simulink model "carry_skip_adder"  (R2022b)
settings: Solver=FixedStepDiscrete  StartTime=0.0  StopTime=10.0  RelTol=1e-3
PreLoadFcn:
  | addpath('C:\Course_Material\UofT\ECE1718\assignment2\matlab_tests\hdlimport\carry_skip_adder');
libraries: simulink x240, hdlsllib x97
(part 1 of 2)
CloseFcn:
  | addpath('C:\Course_Material\UofT\ECE1718\assignment2\matlab_tests\hdlimport\carry_skip_adder');
  | rmpath('C:\Course_Material\UofT\ECE1718\assignment2\matlab_tests\hdlimport\carry_skip_adder');
settings Model: DataTypeOverride=Off  Creator=13698  LastModifiedBy=13698
settings OptimizationCC: BlockReduction=off  ConditionallyExecuteInputs=off  DefaultParameterBehavior=Inlined  InheritOutputTypeSmallerThanSingle=on
settings DebuggingCC: AlgebraicLoopMsg=error  InheritedTsInSrcMsg=none  SingleTaskRateTransMsg=error  IntegerOverflowMsg=none  IntegerSaturationMsg=none
settings HardwareCC: ProdBitPerPointer=32  ProdBitPerSizeT=32  ProdBitPerPtrDiffT=32  ProdLargestAtomicFloat=None  ProdIntDivRoundTo=Undefined  ProdEndianess=Unspecified  ProdWordSize=32  ProdHWDeviceType=ASIC/FPGA->ASIC/FPGA  TargetBitPerPointer=64  TargetBitPerSizeT=64  TargetBitPerPtrDiffT=64  TargetLongLongMode=on  TargetIntDivRoundTo=Zero  TargetEndianess=LittleEndian  TargetWordSize=64  TargetHWDeviceType=Custom Processor->MATLAB Host Computer  ProdEqTarget=off

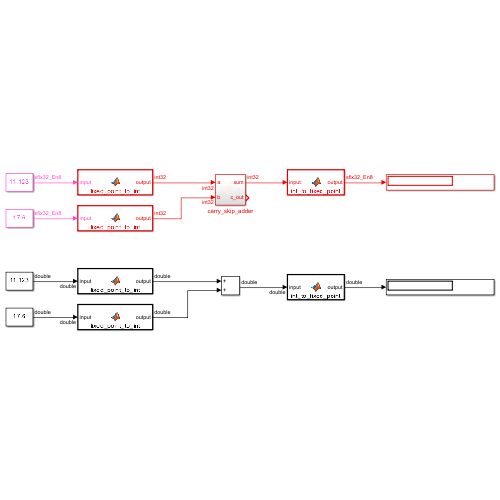
[thumbnail: Simulink's stored preview of the top-level diagram]
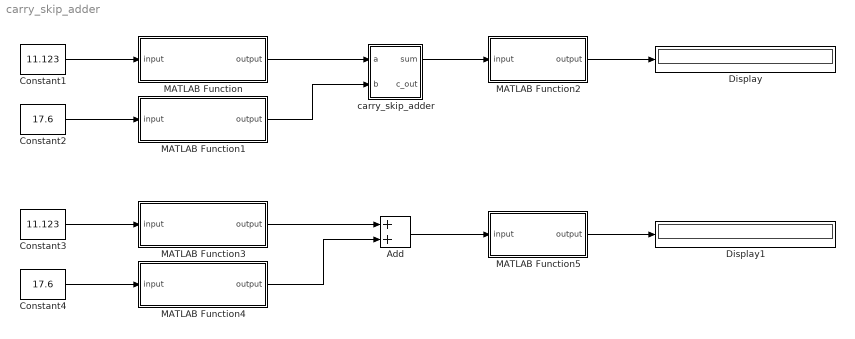
== system carry_skip_adder ==
  Add : Sum
  Constant1 : Constant  Value=11.123  OutDataTypeStr=fixdt(1,32,8)
  Constant2 : Constant  Value=17.6  OutDataTypeStr=fixdt(1,32,8)
  Constant3 : Constant  Value=11.123  OutDataTypeStr=fixdt(1,32,8)
  Constant4 : Constant  Value=17.6  OutDataTypeStr=fixdt(1,32,8)
  Display : Display
  Display1 : Display
  MATLAB Function : MATLAB Function  TreatAsAtomicUnit=on
  MATLAB Function1 : MATLAB Function  TreatAsAtomicUnit=on
  MATLAB Function2 : MATLAB Function  TreatAsAtomicUnit=on
  MATLAB Function3 : MATLAB Function  TreatAsAtomicUnit=on
  MATLAB Function4 : MATLAB Function  TreatAsAtomicUnit=on
  MATLAB Function5 : MATLAB Function  TreatAsAtomicUnit=on
  carry_skip_adder : Subsystem
  wires:
  Constant1/1 -> MATLAB Function/1(input)
  MATLAB Function/1(output) -> carry_skip_adder/1(a)
  Constant2/1 -> MATLAB Function1/1(input)
  MATLAB Function1/1(output) -> carry_skip_adder/2(b)
  carry_skip_adder/1(sum) -> MATLAB Function2/1(input)
  MATLAB Function2/1(output) -> Display/1
  MATLAB Function3/1(output) -> Add/1
  MATLAB Function4/1(output) -> Add/2
  Constant4/1 -> MATLAB Function4/1(input)
  Add/1 -> MATLAB Function5/1(input)
  Constant3/1 -> MATLAB Function3/1(input)
  MATLAB Function5/1(output) -> Display1/1

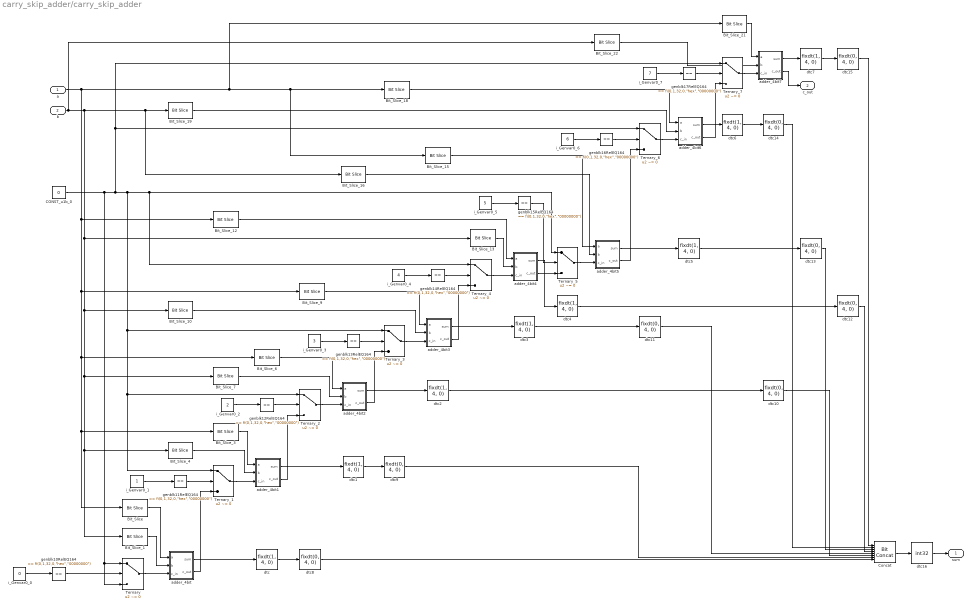
== system carry_skip_adder/carry_skip_adder ==
  a : Inport  OutDataTypeStr=int32  SampleTime=-1
  b : Inport  Port=2  OutDataTypeStr=int32  SampleTime=-1
  Bit_Slice : hdlsllib/Logic and Bit Operations/Bit Slice  lidx=double(3)  ridx=double(0)
  Bit_Slice_1 : hdlsllib/Logic and Bit Operations/Bit Slice  lidx=double(3)  ridx=double(0)
  Bit_Slice_10 : hdlsllib/Logic and Bit Operations/Bit Slice  lidx=double(15)  ridx=double(12)
  Bit_Slice_12 : hdlsllib/Logic and Bit Operations/Bit Slice  lidx=double(19)  ridx=double(16)
  Bit_Slice_13 : hdlsllib/Logic and Bit Operations/Bit Slice  lidx=double(19)  ridx=double(16)
  Bit_Slice_15 : hdlsllib/Logic and Bit Operations/Bit Slice  lidx=double(23)  ridx=double(20)
  Bit_Slice_16 : hdlsllib/Logic and Bit Operations/Bit Slice  lidx=double(23)  ridx=double(20)
  Bit_Slice_18 : hdlsllib/Logic and Bit Operations/Bit Slice  lidx=double(27)  ridx=double(24)
  Bit_Slice_19 : hdlsllib/Logic and Bit Operations/Bit Slice  lidx=double(27)  ridx=double(24)
  Bit_Slice_21 : hdlsllib/Logic and Bit Operations/Bit Slice  lidx=double(31)  ridx=double(28)
  Bit_Slice_22 : hdlsllib/Logic and Bit Operations/Bit Slice  lidx=double(31)  ridx=double(28)
  Bit_Slice_3 : hdlsllib/Logic and Bit Operations/Bit Slice  lidx=double(7)  ridx=double(4)
  Bit_Slice_4 : hdlsllib/Logic and Bit Operations/Bit Slice  lidx=double(7)  ridx=double(4)
  Bit_Slice_6 : hdlsllib/Logic and Bit Operations/Bit Slice  lidx=double(11)  ridx=double(8)
  Bit_Slice_7 : hdlsllib/Logic and Bit Operations/Bit Slice  lidx=double(11)  ridx=double(8)
  Bit_Slice_9 : hdlsllib/Logic and Bit Operations/Bit Slice  lidx=double(15)  ridx=double(12)
  CONST_u1b_0 : Constant  Value=0  OutDataTypeStr=fixdt(0, 1, 0)  SampleTime=-1
  Concat : hdlsllib/Logic and Bit Operations/Bit Concat  numInputs=8
  Ternary : Switch  Criteria=u2 ~= 0  Threshold=double(0)  OutDataTypeStr=fixdt(0, 1, 0)  SampleTime=-1  SaturateOnIntegerOverflow=off  InputSameDT=off
  Ternary_{1..7} (7 alike) : Switch  Criteria=u2 ~= 0  Threshold=double(0)  OutDataTypeStr=fixdt(0, 1, 0)  SampleTime=-1  SaturateOnIntegerOverflow=off  InputSameDT=off
  adder_4bit : Subsystem
  adder_4bit1 : Subsystem
  adder_4bit2 : Subsystem
  adder_4bit3 : Subsystem
  adder_4bit4 : Subsystem
  adder_4bit5 : Subsystem
  adder_4bit6 : Subsystem
  adder_4bit7 : Subsystem
  dtc{,1..7} (8 alike) : DataTypeConversion  OutDataTypeStr=fixdt(1, 4, 0)  SampleTime=-1  SaturateOnIntegerOverflow=off  RndMeth=Floor
  dtc{8..15} (8 alike) : DataTypeConversion  OutDataTypeStr=fixdt(0, 4, 0)  ConvertRealWorld=Stored Integer (SI)  SampleTime=-1  SaturateOnIntegerOverflow=off  RndMeth=Floor
  dtc16 : DataTypeConversion  OutDataTypeStr=int32  ConvertRealWorld=Stored Integer (SI)  SampleTime=-1  SaturateOnIntegerOverflow=off  RndMeth=Floor
  genblk10RelEQ164 : simulink/Logic and Bit Operations/Compare To Constant  relop===  const="fi(0,1,32,0,\"hex\",\"00000000\")"  OutDataTypeStr=boolean
  genblk11RelEQ164 : simulink/Logic and Bit Operations/Compare To Constant  relop===  const="fi(0,1,32,0,\"hex\",\"00000000\")"  OutDataTypeStr=boolean
  genblk12RelEQ164 : simulink/Logic and Bit Operations/Compare To Constant  relop===  const="fi(0,1,32,0,\"hex\",\"00000000\")"  OutDataTypeStr=boolean
  genblk13RelEQ164 : simulink/Logic and Bit Operations/Compare To Constant  relop===  const="fi(0,1,32,0,\"hex\",\"00000000\")"  OutDataTypeStr=boolean
  genblk14RelEQ164 : simulink/Logic and Bit Operations/Compare To Constant  relop===  const="fi(0,1,32,0,\"hex\",\"00000000\")"  OutDataTypeStr=boolean
  genblk15RelEQ164 : simulink/Logic and Bit Operations/Compare To Constant  relop===  const="fi(0,1,32,0,\"hex\",\"00000000\")"  OutDataTypeStr=boolean
  genblk16RelEQ164 : simulink/Logic and Bit Operations/Compare To Constant  relop===  const="fi(0,1,32,0,\"hex\",\"00000000\")"  OutDataTypeStr=boolean
  genblk17RelEQ164 : simulink/Logic and Bit Operations/Compare To Constant  relop===  const="fi(0,1,32,0,\"hex\",\"00000000\")"  OutDataTypeStr=boolean
  i_Genvar0_0 : Constant  Value=0  OutDataTypeStr=int32  SampleTime=-1
  i_Genvar0_1 : Constant  OutDataTypeStr=int32  SampleTime=-1
  i_Genvar0_2 : Constant  Value=2  OutDataTypeStr=int32  SampleTime=-1
  i_Genvar0_3 : Constant  Value=3  OutDataTypeStr=int32  SampleTime=-1
  i_Genvar0_4 : Constant  Value=4  OutDataTypeStr=int32  SampleTime=-1
  i_Genvar0_5 : Constant  Value=5  OutDataTypeStr=int32  SampleTime=-1
  i_Genvar0_6 : Constant  Value=6  OutDataTypeStr=int32  SampleTime=-1
  i_Genvar0_7 : Constant  Value=7  OutDataTypeStr=int32  SampleTime=-1
  sum : Outport  OutDataTypeStr=int32  SampleTime=-1
  c_out : Outport  Port=2  OutDataTypeStr=fixdt(0, 1, 0)  SampleTime=-1
  wires:
  genblk10RelEQ164/1 -> Ternary/2
  Bit_Slice/1 -> adder_4bit/1(a)
  CONST_u1b_0/1 -> Ternary/3, Ternary/1, Ternary_2/1, Ternary_1/1, Ternary_3/1, Ternary_4/1, Ternary_5/1, Ternary_7/1, Ternary_6/1
  adder_4bit3/2(c_out) -> Ternary_4/3
  i_Genvar0_3/1 -> genblk13RelEQ164/1
  i_Genvar0_0/1 -> genblk10RelEQ164/1
  dtc2/1 -> dtc10/1
  i_Genvar0_1/1 -> genblk11RelEQ164/1
  genblk15RelEQ164/1 -> Ternary_5/2
  Bit_Slice_12/1 -> adder_4bit4/1(a)
  adder_4bit3/1(sum) -> dtc3/1
  a/1 -> Bit_Slice_3/1, Bit_Slice/1, Bit_Slice_6/1, Bit_Slice_9/1, Bit_Slice_12/1, Bit_Slice_15/1, Bit_Slice_18/1, Bit_Slice_21/1
  b/1 -> Bit_Slice_4/1, Bit_Slice_1/1, Bit_Slice_7/1, Bit_Slice_10/1, Bit_Slice_13/1, Bit_Slice_19/1, Bit_Slice_16/1, Bit_Slice_22/1
  dtc4/1 -> dtc12/1
  dtc1/1 -> dtc9/1
  Bit_Slice_1/1 -> adder_4bit/2(b)
  Ternary_6/1 -> adder_4bit6/3(c_in)
  Ternary/1 -> adder_4bit/3(c_in)
  Bit_Slice_19/1 -> adder_4bit6/2(b)
  adder_4bit5/2(c_out) -> Ternary_6/3
  adder_4bit4/1(sum) -> dtc4/1
  Bit_Slice_10/1 -> adder_4bit3/2(b)
  Bit_Slice_4/1 -> adder_4bit1/2(b)
  adder_4bit5/1(sum) -> dtc5/1
  Bit_Slice_7/1 -> adder_4bit2/2(b)
  genblk11RelEQ164/1 -> Ternary_1/2
  adder_4bit/1(sum) -> dtc/1
  adder_4bit/2(c_out) -> Ternary_1/3
  i_Genvar0_2/1 -> genblk12RelEQ164/1
  i_Genvar0_4/1 -> genblk14RelEQ164/1
  adder_4bit1/1(sum) -> dtc1/1
  Bit_Slice_3/1 -> adder_4bit1/1(a)
  Bit_Slice_16/1 -> adder_4bit5/2(b)
  Ternary_1/1 -> adder_4bit1/3(c_in)
  genblk13RelEQ164/1 -> Ternary_3/2
  Bit_Slice_6/1 -> adder_4bit2/1(a)
  genblk12RelEQ164/1 -> Ternary_2/2
  adder_4bit1/2(c_out) -> Ternary_2/3
  dtc/1 -> dtc8/1
  dtc11/1 -> Concat/5
  genblk14RelEQ164/1 -> Ternary_4/2
  Bit_Slice_9/1 -> adder_4bit3/1(a)
  i_Genvar0_6/1 -> genblk16RelEQ164/1
  Ternary_2/1 -> adder_4bit2/3(c_in)
  Ternary_4/1 -> adder_4bit4/3(c_in)
  dtc8/1 -> Concat/8
  adder_4bit2/1(sum) -> dtc2/1
  adder_4bit2/2(c_out) -> Ternary_3/3
  genblk17RelEQ164/1 -> Ternary_7/2
  Bit_Slice_18/1 -> adder_4bit6/1(a)
  i_Genvar0_7/1 -> genblk17RelEQ164/1
  Ternary_3/1 -> adder_4bit3/3(c_in)
  dtc9/1 -> Concat/7
  genblk16RelEQ164/1 -> Ternary_6/2
  Bit_Slice_15/1 -> adder_4bit5/1(a)
  i_Genvar0_5/1 -> genblk15RelEQ164/1
  Bit_Slice_13/1 -> adder_4bit4/2(b)
  adder_4bit4/2(c_out) -> Ternary_5/3
  dtc3/1 -> dtc11/1
  Ternary_5/1 -> adder_4bit5/3(c_in)
  Bit_Slice_22/1 -> adder_4bit7/2(b)
  adder_4bit6/1(sum) -> dtc6/1
  adder_4bit6/2(c_out) -> Ternary_7/3
  dtc5/1 -> dtc13/1
  Bit_Slice_21/1 -> adder_4bit7/1(a)
  Ternary_7/1 -> adder_4bit7/3(c_in)
  dtc6/1 -> dtc14/1
  adder_4bit7/1(sum) -> dtc7/1
  adder_4bit7/2(c_out) -> c_out/1
  dtc14/1 -> Concat/2
  dtc10/1 -> Concat/6
  dtc7/1 -> dtc15/1
  dtc13/1 -> Concat/3
  dtc15/1 -> Concat/1
  dtc12/1 -> Concat/4
  Concat/1 -> dtc16/1
  dtc16/1 -> sum/1

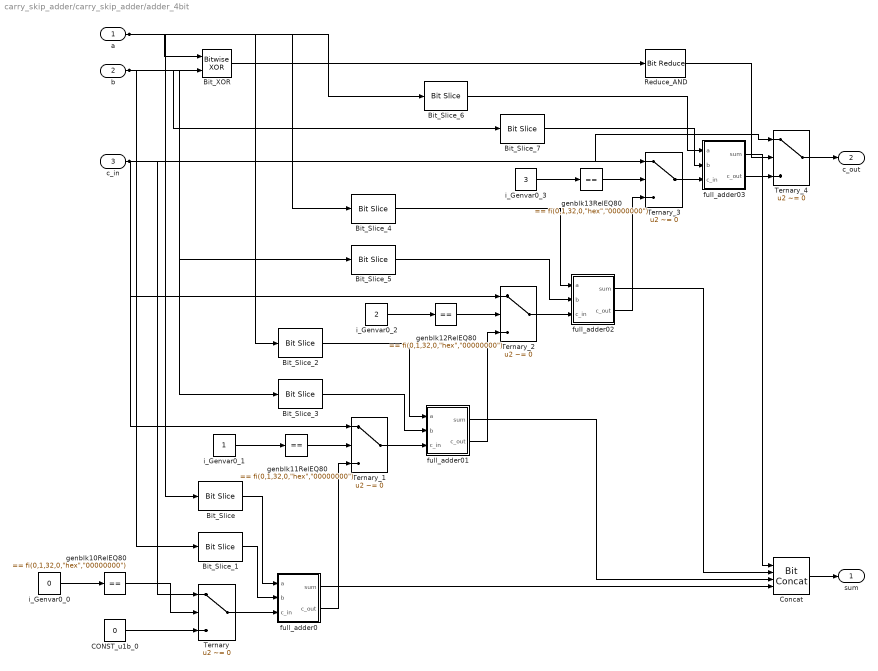
== system carry_skip_adder/carry_skip_adder/adder_4bit ==
  a : Inport  OutDataTypeStr=fixdt(0, 4, 0)  SampleTime=-1
  b : Inport  Port=2  OutDataTypeStr=fixdt(0, 4, 0)  SampleTime=-1
  c_in : Inport  Port=3  OutDataTypeStr=fixdt(0, 1, 0)  SampleTime=-1
  Bit_Slice : hdlsllib/Logic and Bit Operations/Bit Slice  lidx=double(0)  ridx=double(0)
  Bit_Slice_1 : hdlsllib/Logic and Bit Operations/Bit Slice  lidx=double(0)  ridx=double(0)
  Bit_Slice_2 : hdlsllib/Logic and Bit Operations/Bit Slice  lidx=double(1)  ridx=double(1)
  Bit_Slice_3 : hdlsllib/Logic and Bit Operations/Bit Slice  lidx=double(1)  ridx=double(1)
  Bit_Slice_4 : hdlsllib/Logic and Bit Operations/Bit Slice  lidx=double(2)  ridx=double(2)
  Bit_Slice_5 : hdlsllib/Logic and Bit Operations/Bit Slice  lidx=double(2)  ridx=double(2)
  Bit_Slice_6 : hdlsllib/Logic and Bit Operations/Bit Slice  lidx=double(3)  ridx=double(3)
  Bit_Slice_7 : hdlsllib/Logic and Bit Operations/Bit Slice  lidx=double(3)  ridx=double(3)
  Bit_XOR : simulink/Logic and Bit Operations/Bitwise Operator  logicop=XOR  UseBitMask=off  NumInputPorts=2  BitMask=double(0)  BitMaskRealWorld=Real World Value
  CONST_u1b_0 : Constant  Value=0  OutDataTypeStr=fixdt(0, 1, 0)  SampleTime=-1
  Concat : hdlsllib/Logic and Bit Operations/Bit Concat  numInputs=4
  Reduce_AND : hdlsllib/Logic and Bit Operations/Bit Reduce  mode=AND
  Ternary : Switch  Criteria=u2 ~= 0  Threshold=double(0)  OutDataTypeStr=fixdt(0, 1, 0)  SampleTime=-1  SaturateOnIntegerOverflow=off  InputSameDT=off
  Ternary_{1..4} (4 alike) : Switch  Criteria=u2 ~= 0  Threshold=double(0)  OutDataTypeStr=fixdt(0, 1, 0)  SampleTime=-1  SaturateOnIntegerOverflow=off  InputSameDT=off
  full_adder0 : Subsystem
  full_adder01 : Subsystem
  full_adder02 : Subsystem
  full_adder03 : Subsystem
  genblk10RelEQ80 : simulink/Logic and Bit Operations/Compare To Constant  relop===  const="fi(0,1,32,0,\"hex\",\"00000000\")"  OutDataTypeStr=boolean
  genblk11RelEQ80 : simulink/Logic and Bit Operations/Compare To Constant  relop===  const="fi(0,1,32,0,\"hex\",\"00000000\")"  OutDataTypeStr=boolean
  genblk12RelEQ80 : simulink/Logic and Bit Operations/Compare To Constant  relop===  const="fi(0,1,32,0,\"hex\",\"00000000\")"  OutDataTypeStr=boolean
  genblk13RelEQ80 : simulink/Logic and Bit Operations/Compare To Constant  relop===  const="fi(0,1,32,0,\"hex\",\"00000000\")"  OutDataTypeStr=boolean
  i_Genvar0_0 : Constant  Value=0  OutDataTypeStr=int32  SampleTime=-1
  i_Genvar0_1 : Constant  OutDataTypeStr=int32  SampleTime=-1
  i_Genvar0_2 : Constant  Value=2  OutDataTypeStr=int32  SampleTime=-1
  i_Genvar0_3 : Constant  Value=3  OutDataTypeStr=int32  SampleTime=-1
  sum : Outport  OutDataTypeStr=fixdt(0, 4, 0)  SampleTime=-1
  c_out : Outport  Port=2  OutDataTypeStr=fixdt(0, 1, 0)  SampleTime=-1
  wires:
  full_adder03/2(c_out) -> Ternary_4/3
  i_Genvar0_0/1 -> genblk10RelEQ80/1
  Bit_Slice_7/1 -> full_adder03/2(b)
  full_adder0/2(c_out) -> Ternary_1/3
  a/1 -> Bit_Slice_4/1, Bit_Slice_2/1, Bit_Slice/1, Bit_Slice_6/1, Bit_XOR/1
  b/1 -> Bit_Slice_3/1, Bit_Slice_7/1, Bit_Slice_1/1, Bit_Slice_5/1, Bit_XOR/2
  Bit_XOR/1 -> Reduce_AND/1
  CONST_u1b_0/1 -> Ternary/3
  Ternary_3/1 -> full_adder03/3(c_in)
  c_in/1 -> Ternary_4/1, Ternary_1/1, Ternary_3/1, Ternary_2/1, Ternary/1
  i_Genvar0_1/1 -> genblk11RelEQ80/1
  genblk10RelEQ80/1 -> Ternary/2
  Bit_Slice/1 -> full_adder0/1(a)
  Bit_Slice_5/1 -> full_adder02/2(b)
  Bit_Slice_1/1 -> full_adder0/2(b)
  Ternary/1 -> full_adder0/3(c_in)
  Bit_Slice_2/1 -> full_adder01/1(a)
  Bit_Slice_3/1 -> full_adder01/2(b)
  genblk11RelEQ80/1 -> Ternary_1/2
  full_adder0/1(sum) -> Concat/4
  full_adder02/2(c_out) -> Ternary_3/3
  Bit_Slice_4/1 -> full_adder02/1(a)
  i_Genvar0_2/1 -> genblk12RelEQ80/1
  Ternary_1/1 -> full_adder01/3(c_in)
  Bit_Slice_6/1 -> full_adder03/1(a)
  genblk12RelEQ80/1 -> Ternary_2/2
  full_adder01/1(sum) -> Concat/3
  full_adder01/2(c_out) -> Ternary_2/3
  i_Genvar0_3/1 -> genblk13RelEQ80/1
  full_adder03/1(sum) -> Concat/1
  Ternary_2/1 -> full_adder02/3(c_in)
  Concat/1 -> sum/1
  genblk13RelEQ80/1 -> Ternary_3/2
  full_adder02/1(sum) -> Concat/2
  Reduce_AND/1 -> Ternary_4/2
  Ternary_4/1 -> c_out/1

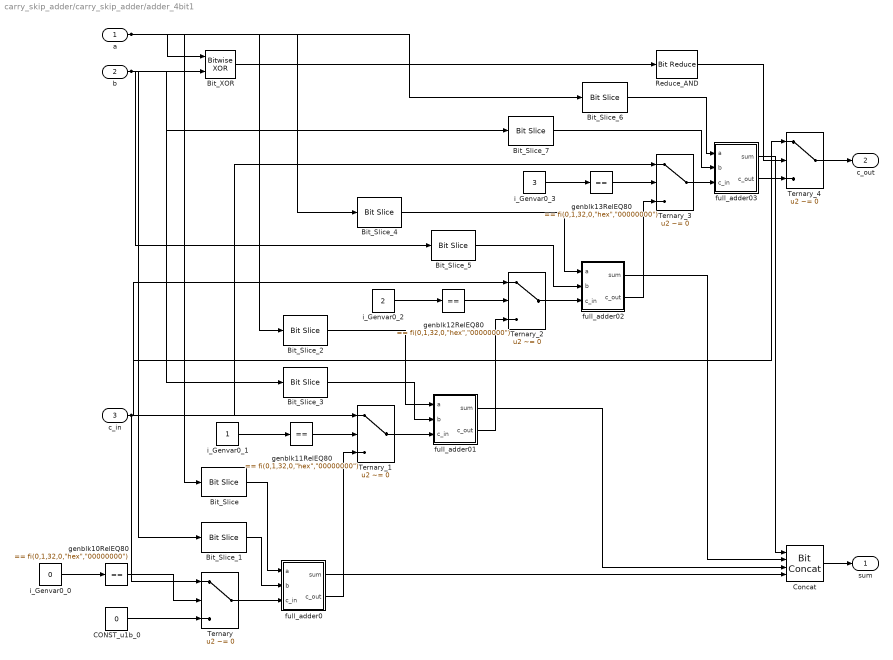
== system carry_skip_adder/carry_skip_adder/adder_4bit1 ==
  a : Inport  OutDataTypeStr=fixdt(0, 4, 0)  SampleTime=-1
  b : Inport  Port=2  OutDataTypeStr=fixdt(0, 4, 0)  SampleTime=-1
  c_in : Inport  Port=3  OutDataTypeStr=fixdt(0, 1, 0)  SampleTime=-1
  Bit_Slice : hdlsllib/Logic and Bit Operations/Bit Slice  lidx=double(0)  ridx=double(0)
  Bit_Slice_1 : hdlsllib/Logic and Bit Operations/Bit Slice  lidx=double(0)  ridx=double(0)
  Bit_Slice_2 : hdlsllib/Logic and Bit Operations/Bit Slice  lidx=double(1)  ridx=double(1)
  Bit_Slice_3 : hdlsllib/Logic and Bit Operations/Bit Slice  lidx=double(1)  ridx=double(1)
  Bit_Slice_4 : hdlsllib/Logic and Bit Operations/Bit Slice  lidx=double(2)  ridx=double(2)
  Bit_Slice_5 : hdlsllib/Logic and Bit Operations/Bit Slice  lidx=double(2)  ridx=double(2)
  Bit_Slice_6 : hdlsllib/Logic and Bit Operations/Bit Slice  lidx=double(3)  ridx=double(3)
  Bit_Slice_7 : hdlsllib/Logic and Bit Operations/Bit Slice  lidx=double(3)  ridx=double(3)
  Bit_XOR : simulink/Logic and Bit Operations/Bitwise Operator  logicop=XOR  UseBitMask=off  NumInputPorts=2  BitMask=double(0)  BitMaskRealWorld=Real World Value
  CONST_u1b_0 : Constant  Value=0  OutDataTypeStr=fixdt(0, 1, 0)  SampleTime=-1
  Concat : hdlsllib/Logic and Bit Operations/Bit Concat  numInputs=4
  Reduce_AND : hdlsllib/Logic and Bit Operations/Bit Reduce  mode=AND
  Ternary : Switch  Criteria=u2 ~= 0  Threshold=double(0)  OutDataTypeStr=fixdt(0, 1, 0)  SampleTime=-1  SaturateOnIntegerOverflow=off  InputSameDT=off
  Ternary_{1..4} (4 alike) : Switch  Criteria=u2 ~= 0  Threshold=double(0)  OutDataTypeStr=fixdt(0, 1, 0)  SampleTime=-1  SaturateOnIntegerOverflow=off  InputSameDT=off
  full_adder0 : Subsystem
  full_adder01 : Subsystem
  full_adder02 : Subsystem
  full_adder03 : Subsystem
  genblk10RelEQ80 : simulink/Logic and Bit Operations/Compare To Constant  relop===  const="fi(0,1,32,0,\"hex\",\"00000000\")"  OutDataTypeStr=boolean
  genblk11RelEQ80 : simulink/Logic and Bit Operations/Compare To Constant  relop===  const="fi(0,1,32,0,\"hex\",\"00000000\")"  OutDataTypeStr=boolean
  genblk12RelEQ80 : simulink/Logic and Bit Operations/Compare To Constant  relop===  const="fi(0,1,32,0,\"hex\",\"00000000\")"  OutDataTypeStr=boolean
  genblk13RelEQ80 : simulink/Logic and Bit Operations/Compare To Constant  relop===  const="fi(0,1,32,0,\"hex\",\"00000000\")"  OutDataTypeStr=boolean
  i_Genvar0_0 : Constant  Value=0  OutDataTypeStr=int32  SampleTime=-1
  i_Genvar0_1 : Constant  OutDataTypeStr=int32  SampleTime=-1
  i_Genvar0_2 : Constant  Value=2  OutDataTypeStr=int32  SampleTime=-1
  i_Genvar0_3 : Constant  Value=3  OutDataTypeStr=int32  SampleTime=-1
  sum : Outport  OutDataTypeStr=fixdt(0, 4, 0)  SampleTime=-1
  c_out : Outport  Port=2  OutDataTypeStr=fixdt(0, 1, 0)  SampleTime=-1
  wires:
  Ternary_4/1 -> c_out/1
  i_Genvar0_0/1 -> genblk10RelEQ80/1
  a/1 -> Bit_Slice_6/1, Bit_Slice_2/1, Bit_Slice/1, Bit_XOR/1, Bit_Slice_4/1
  genblk10RelEQ80/1 -> Ternary/2
  b/1 -> Bit_Slice_7/1, Bit_Slice_5/1, Bit_Slice_1/1, Bit_Slice_3/1, Bit_XOR/2
  genblk13RelEQ80/1 -> Ternary_3/2
  Bit_Slice_6/1 -> full_adder03/1(a)
  full_adder01/2(c_out) -> Ternary_2/3
  Bit_XOR/1 -> Reduce_AND/1
  Ternary_1/1 -> full_adder01/3(c_in)
  CONST_u1b_0/1 -> Ternary/3
  c_in/1 -> Ternary_2/1, Ternary_4/1, Ternary_1/1, Ternary_3/1, Ternary/1
  i_Genvar0_1/1 -> genblk11RelEQ80/1
  Bit_Slice/1 -> full_adder0/1(a)
  Bit_Slice_1/1 -> full_adder0/2(b)
  Ternary/1 -> full_adder0/3(c_in)
  Bit_Slice_2/1 -> full_adder01/1(a)
  Bit_Slice_3/1 -> full_adder01/2(b)
  genblk11RelEQ80/1 -> Ternary_1/2
  full_adder0/1(sum) -> Concat/4
  full_adder0/2(c_out) -> Ternary_1/3
  Bit_Slice_4/1 -> full_adder02/1(a)
  i_Genvar0_2/1 -> genblk12RelEQ80/1
  Bit_Slice_5/1 -> full_adder02/2(b)
  genblk12RelEQ80/1 -> Ternary_2/2
  full_adder01/1(sum) -> Concat/3
  Bit_Slice_7/1 -> full_adder03/2(b)
  Concat/1 -> sum/1
  i_Genvar0_3/1 -> genblk13RelEQ80/1
  Reduce_AND/1 -> Ternary_4/2
  Ternary_2/1 -> full_adder02/3(c_in)
  full_adder03/1(sum) -> Concat/1
  full_adder02/1(sum) -> Concat/2
  full_adder02/2(c_out) -> Ternary_3/3
  Ternary_3/1 -> full_adder03/3(c_in)
  full_adder03/2(c_out) -> Ternary_4/3

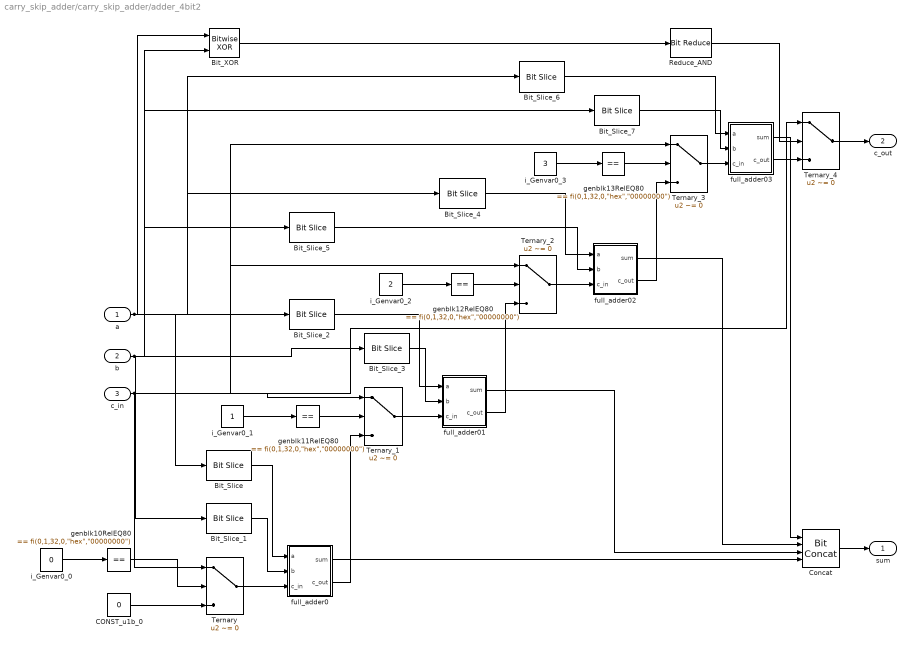
== system carry_skip_adder/carry_skip_adder/adder_4bit2 ==
  a : Inport  OutDataTypeStr=fixdt(0, 4, 0)  SampleTime=-1
  b : Inport  Port=2  OutDataTypeStr=fixdt(0, 4, 0)  SampleTime=-1
  c_in : Inport  Port=3  OutDataTypeStr=fixdt(0, 1, 0)  SampleTime=-1
  Bit_Slice : hdlsllib/Logic and Bit Operations/Bit Slice  lidx=double(0)  ridx=double(0)
  Bit_Slice_1 : hdlsllib/Logic and Bit Operations/Bit Slice  lidx=double(0)  ridx=double(0)
  Bit_Slice_2 : hdlsllib/Logic and Bit Operations/Bit Slice  lidx=double(1)  ridx=double(1)
  Bit_Slice_3 : hdlsllib/Logic and Bit Operations/Bit Slice  lidx=double(1)  ridx=double(1)
  Bit_Slice_4 : hdlsllib/Logic and Bit Operations/Bit Slice  lidx=double(2)  ridx=double(2)
  Bit_Slice_5 : hdlsllib/Logic and Bit Operations/Bit Slice  lidx=double(2)  ridx=double(2)
  Bit_Slice_6 : hdlsllib/Logic and Bit Operations/Bit Slice  lidx=double(3)  ridx=double(3)
  Bit_Slice_7 : hdlsllib/Logic and Bit Operations/Bit Slice  lidx=double(3)  ridx=double(3)
  Bit_XOR : simulink/Logic and Bit Operations/Bitwise Operator  logicop=XOR  UseBitMask=off  NumInputPorts=2  BitMask=double(0)  BitMaskRealWorld=Real World Value
  CONST_u1b_0 : Constant  Value=0  OutDataTypeStr=fixdt(0, 1, 0)  SampleTime=-1
  Concat : hdlsllib/Logic and Bit Operations/Bit Concat  numInputs=4
  Reduce_AND : hdlsllib/Logic and Bit Operations/Bit Reduce  mode=AND
  Ternary : Switch  Criteria=u2 ~= 0  Threshold=double(0)  OutDataTypeStr=fixdt(0, 1, 0)  SampleTime=-1  SaturateOnIntegerOverflow=off  InputSameDT=off
  Ternary_{1..4} (4 alike) : Switch  Criteria=u2 ~= 0  Threshold=double(0)  OutDataTypeStr=fixdt(0, 1, 0)  SampleTime=-1  SaturateOnIntegerOverflow=off  InputSameDT=off
  full_adder0 : Subsystem
  full_adder01 : Subsystem
  full_adder02 : Subsystem
  full_adder03 : Subsystem
  genblk10RelEQ80 : simulink/Logic and Bit Operations/Compare To Constant  relop===  const="fi(0,1,32,0,\"hex\",\"00000000\")"  OutDataTypeStr=boolean
  genblk11RelEQ80 : simulink/Logic and Bit Operations/Compare To Constant  relop===  const="fi(0,1,32,0,\"hex\",\"00000000\")"  OutDataTypeStr=boolean
  genblk12RelEQ80 : simulink/Logic and Bit Operations/Compare To Constant  relop===  const="fi(0,1,32,0,\"hex\",\"00000000\")"  OutDataTypeStr=boolean
  genblk13RelEQ80 : simulink/Logic and Bit Operations/Compare To Constant  relop===  const="fi(0,1,32,0,\"hex\",\"00000000\")"  OutDataTypeStr=boolean
  i_Genvar0_0 : Constant  Value=0  OutDataTypeStr=int32  SampleTime=-1
  i_Genvar0_1 : Constant  OutDataTypeStr=int32  SampleTime=-1
  i_Genvar0_2 : Constant  Value=2  OutDataTypeStr=int32  SampleTime=-1
  i_Genvar0_3 : Constant  Value=3  OutDataTypeStr=int32  SampleTime=-1
  sum : Outport  OutDataTypeStr=fixdt(0, 4, 0)  SampleTime=-1
  c_out : Outport  Port=2  OutDataTypeStr=fixdt(0, 1, 0)  SampleTime=-1
  wires:
  i_Genvar0_0/1 -> genblk10RelEQ80/1
  a/1 -> Bit_Slice_6/1, Bit_Slice_4/1, Bit_Slice_2/1, Bit_XOR/1, Bit_Slice/1
  Bit_XOR/1 -> Reduce_AND/1
  b/1 -> Bit_Slice_7/1, Bit_Slice_5/1, Bit_Slice_1/1, Bit_XOR/2, Bit_Slice_3/1
  c_in/1 -> Ternary_4/1, Ternary_3/1, Ternary_2/1, Ternary_1/1, Ternary/1
  genblk10RelEQ80/1 -> Ternary/2
  full_adder0/2(c_out) -> Ternary_1/3
  i_Genvar0_1/1 -> genblk11RelEQ80/1
  CONST_u1b_0/1 -> Ternary/3
  Bit_Slice/1 -> full_adder0/1(a)
  full_adder02/2(c_out) -> Ternary_3/3
  Bit_Slice_1/1 -> full_adder0/2(b)
  i_Genvar0_2/1 -> genblk12RelEQ80/1
  Ternary/1 -> full_adder0/3(c_in)
  Bit_Slice_5/1 -> full_adder02/2(b)
  Bit_Slice_2/1 -> full_adder01/1(a)
  genblk11RelEQ80/1 -> Ternary_1/2
  full_adder0/1(sum) -> Concat/4
  Bit_Slice_3/1 -> full_adder01/2(b)
  Ternary_1/1 -> full_adder01/3(c_in)
  full_adder03/2(c_out) -> Ternary_4/3
  Bit_Slice_4/1 -> full_adder02/1(a)
  genblk12RelEQ80/1 -> Ternary_2/2
  full_adder01/1(sum) -> Concat/3
  full_adder01/2(c_out) -> Ternary_2/3
  Bit_Slice_6/1 -> full_adder03/1(a)
  i_Genvar0_3/1 -> genblk13RelEQ80/1
  Reduce_AND/1 -> Ternary_4/2
  Ternary_2/1 -> full_adder02/3(c_in)
  Bit_Slice_7/1 -> full_adder03/2(b)
  full_adder03/1(sum) -> Concat/1
  genblk13RelEQ80/1 -> Ternary_3/2
  full_adder02/1(sum) -> Concat/2
  Ternary_3/1 -> full_adder03/3(c_in)
  Concat/1 -> sum/1
  Ternary_4/1 -> c_out/1

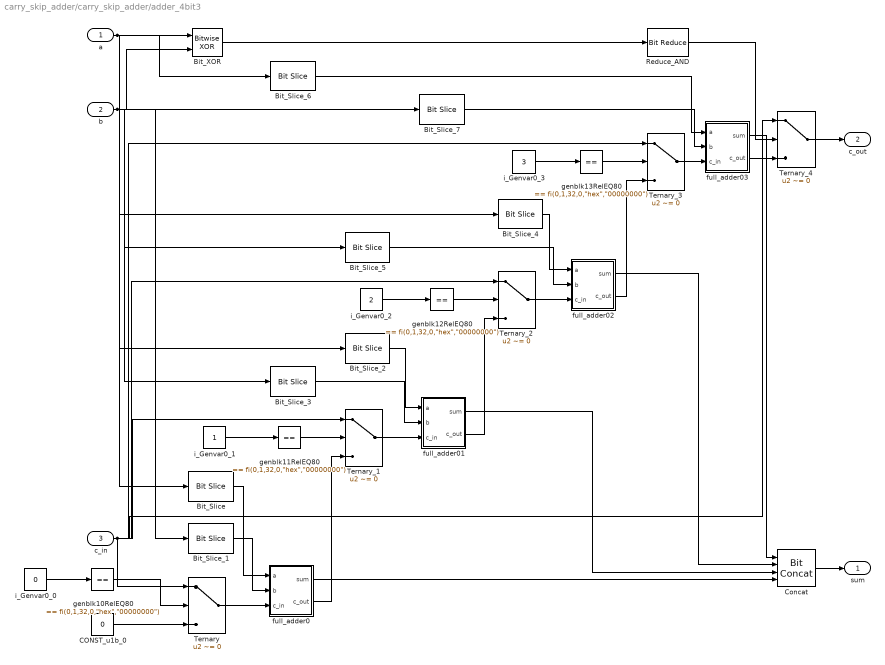
== system carry_skip_adder/carry_skip_adder/adder_4bit3 ==
  a : Inport  OutDataTypeStr=fixdt(0, 4, 0)  SampleTime=-1
  b : Inport  Port=2  OutDataTypeStr=fixdt(0, 4, 0)  SampleTime=-1
  c_in : Inport  Port=3  OutDataTypeStr=fixdt(0, 1, 0)  SampleTime=-1
  Bit_Slice : hdlsllib/Logic and Bit Operations/Bit Slice  lidx=double(0)  ridx=double(0)
  Bit_Slice_1 : hdlsllib/Logic and Bit Operations/Bit Slice  lidx=double(0)  ridx=double(0)
  Bit_Slice_2 : hdlsllib/Logic and Bit Operations/Bit Slice  lidx=double(1)  ridx=double(1)
  Bit_Slice_3 : hdlsllib/Logic and Bit Operations/Bit Slice  lidx=double(1)  ridx=double(1)
  Bit_Slice_4 : hdlsllib/Logic and Bit Operations/Bit Slice  lidx=double(2)  ridx=double(2)
  Bit_Slice_5 : hdlsllib/Logic and Bit Operations/Bit Slice  lidx=double(2)  ridx=double(2)
  Bit_Slice_6 : hdlsllib/Logic and Bit Operations/Bit Slice  lidx=double(3)  ridx=double(3)
  Bit_Slice_7 : hdlsllib/Logic and Bit Operations/Bit Slice  lidx=double(3)  ridx=double(3)
  Bit_XOR : simulink/Logic and Bit Operations/Bitwise Operator  logicop=XOR  UseBitMask=off  NumInputPorts=2  BitMask=double(0)  BitMaskRealWorld=Real World Value
  CONST_u1b_0 : Constant  Value=0  OutDataTypeStr=fixdt(0, 1, 0)  SampleTime=-1
  Concat : hdlsllib/Logic and Bit Operations/Bit Concat  numInputs=4
  Reduce_AND : hdlsllib/Logic and Bit Operations/Bit Reduce  mode=AND
  Ternary : Switch  Criteria=u2 ~= 0  Threshold=double(0)  OutDataTypeStr=fixdt(0, 1, 0)  SampleTime=-1  SaturateOnIntegerOverflow=off  InputSameDT=off
  Ternary_{1..4} (4 alike) : Switch  Criteria=u2 ~= 0  Threshold=double(0)  OutDataTypeStr=fixdt(0, 1, 0)  SampleTime=-1  SaturateOnIntegerOverflow=off  InputSameDT=off
  full_adder0 : Subsystem
  full_adder01 : Subsystem
  full_adder02 : Subsystem
  full_adder03 : Subsystem
  genblk10RelEQ80 : simulink/Logic and Bit Operations/Compare To Constant  relop===  const="fi(0,1,32,0,\"hex\",\"00000000\")"  OutDataTypeStr=boolean
  genblk11RelEQ80 : simulink/Logic and Bit Operations/Compare To Constant  relop===  const="fi(0,1,32,0,\"hex\",\"00000000\")"  OutDataTypeStr=boolean
  genblk12RelEQ80 : simulink/Logic and Bit Operations/Compare To Constant  relop===  const="fi(0,1,32,0,\"hex\",\"00000000\")"  OutDataTypeStr=boolean
  genblk13RelEQ80 : simulink/Logic and Bit Operations/Compare To Constant  relop===  const="fi(0,1,32,0,\"hex\",\"00000000\")"  OutDataTypeStr=boolean
  i_Genvar0_0 : Constant  Value=0  OutDataTypeStr=int32  SampleTime=-1
  i_Genvar0_1 : Constant  OutDataTypeStr=int32  SampleTime=-1
  i_Genvar0_2 : Constant  Value=2  OutDataTypeStr=int32  SampleTime=-1
  i_Genvar0_3 : Constant  Value=3  OutDataTypeStr=int32  SampleTime=-1
  sum : Outport  OutDataTypeStr=fixdt(0, 4, 0)  SampleTime=-1
  c_out : Outport  Port=2  OutDataTypeStr=fixdt(0, 1, 0)  SampleTime=-1
  wires:
  i_Genvar0_3/1 -> genblk13RelEQ80/1
  a/1 -> Bit_Slice_4/1, Bit_Slice_6/1, Bit_Slice_2/1, Bit_Slice/1, Bit_XOR/1
  i_Genvar0_0/1 -> genblk10RelEQ80/1
  Bit_XOR/1 -> Reduce_AND/1
  b/1 -> Bit_Slice_7/1, Bit_Slice_5/1, Bit_Slice_1/1, Bit_Slice_3/1, Bit_XOR/2
  CONST_u1b_0/1 -> Ternary/3
  c_in/1 -> Ternary_4/1, Ternary_3/1, Ternary_2/1, Ternary_1/1, Ternary/1
  genblk10RelEQ80/1 -> Ternary/2
  i_Genvar0_1/1 -> genblk11RelEQ80/1
  Bit_Slice/1 -> full_adder0/1(a)
  Bit_Slice_7/1 -> full_adder03/2(b)
  Bit_Slice_1/1 -> full_adder0/2(b)
  i_Genvar0_2/1 -> genblk12RelEQ80/1
  Ternary/1 -> full_adder0/3(c_in)
  full_adder02/2(c_out) -> Ternary_3/3
  genblk11RelEQ80/1 -> Ternary_1/2
  Bit_Slice_6/1 -> full_adder03/1(a)
  full_adder0/1(sum) -> Concat/4
  Bit_Slice_3/1 -> full_adder01/2(b)
  full_adder02/1(sum) -> Concat/2
  full_adder0/2(c_out) -> Ternary_1/3
  Bit_Slice_5/1 -> full_adder02/2(b)
  Bit_Slice_2/1 -> full_adder01/1(a)
  Ternary_1/1 -> full_adder01/3(c_in)
  genblk12RelEQ80/1 -> Ternary_2/2
  full_adder01/1(sum) -> Concat/3
  Ternary_3/1 -> full_adder03/3(c_in)
  full_adder01/2(c_out) -> Ternary_2/3
  Bit_Slice_4/1 -> full_adder02/1(a)
  Reduce_AND/1 -> Ternary_4/2
  Ternary_2/1 -> full_adder02/3(c_in)
  genblk13RelEQ80/1 -> Ternary_3/2
  full_adder03/1(sum) -> Concat/1
  full_adder03/2(c_out) -> Ternary_4/3
  Ternary_4/1 -> c_out/1
  Concat/1 -> sum/1

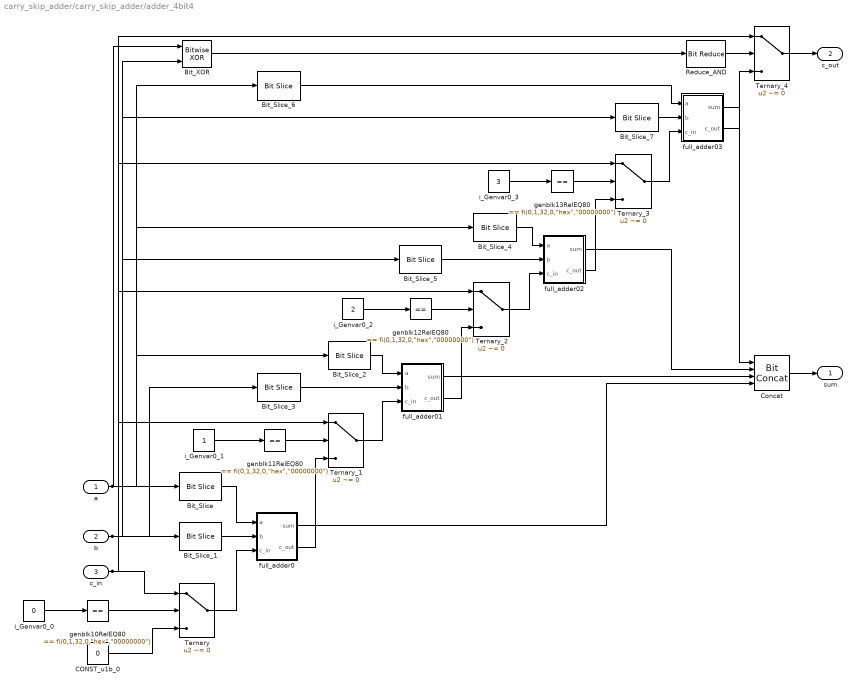
== system carry_skip_adder/carry_skip_adder/adder_4bit4 ==
  a : Inport  OutDataTypeStr=fixdt(0, 4, 0)  SampleTime=-1
  b : Inport  Port=2  OutDataTypeStr=fixdt(0, 4, 0)  SampleTime=-1
  c_in : Inport  Port=3  OutDataTypeStr=fixdt(0, 1, 0)  SampleTime=-1
  Bit_Slice : hdlsllib/Logic and Bit Operations/Bit Slice  lidx=double(0)  ridx=double(0)
  Bit_Slice_1 : hdlsllib/Logic and Bit Operations/Bit Slice  lidx=double(0)  ridx=double(0)
  Bit_Slice_2 : hdlsllib/Logic and Bit Operations/Bit Slice  lidx=double(1)  ridx=double(1)
  Bit_Slice_3 : hdlsllib/Logic and Bit Operations/Bit Slice  lidx=double(1)  ridx=double(1)
  Bit_Slice_4 : hdlsllib/Logic and Bit Operations/Bit Slice  lidx=double(2)  ridx=double(2)
  Bit_Slice_5 : hdlsllib/Logic and Bit Operations/Bit Slice  lidx=double(2)  ridx=double(2)
  Bit_Slice_6 : hdlsllib/Logic and Bit Operations/Bit Slice  lidx=double(3)  ridx=double(3)
  Bit_Slice_7 : hdlsllib/Logic and Bit Operations/Bit Slice  lidx=double(3)  ridx=double(3)
  Bit_XOR : simulink/Logic and Bit Operations/Bitwise Operator  logicop=XOR  UseBitMask=off  NumInputPorts=2  BitMask=double(0)  BitMaskRealWorld=Real World Value
  CONST_u1b_0 : Constant  Value=0  OutDataTypeStr=fixdt(0, 1, 0)  SampleTime=-1
  Concat : hdlsllib/Logic and Bit Operations/Bit Concat  numInputs=4
  Reduce_AND : hdlsllib/Logic and Bit Operations/Bit Reduce  mode=AND
  Ternary : Switch  Criteria=u2 ~= 0  Threshold=double(0)  OutDataTypeStr=fixdt(0, 1, 0)  SampleTime=-1  SaturateOnIntegerOverflow=off  InputSameDT=off
  Ternary_{1..4} (4 alike) : Switch  Criteria=u2 ~= 0  Threshold=double(0)  OutDataTypeStr=fixdt(0, 1, 0)  SampleTime=-1  SaturateOnIntegerOverflow=off  InputSameDT=off
  full_adder0 : Subsystem
  full_adder01 : Subsystem
  full_adder02 : Subsystem
  full_adder03 : Subsystem
  genblk10RelEQ80 : simulink/Logic and Bit Operations/Compare To Constant  relop===  const="fi(0,1,32,0,\"hex\",\"00000000\")"  OutDataTypeStr=boolean
  genblk11RelEQ80 : simulink/Logic and Bit Operations/Compare To Constant  relop===  const="fi(0,1,32,0,\"hex\",\"00000000\")"  OutDataTypeStr=boolean
  genblk12RelEQ80 : simulink/Logic and Bit Operations/Compare To Constant  relop===  const="fi(0,1,32,0,\"hex\",\"00000000\")"  OutDataTypeStr=boolean
  genblk13RelEQ80 : simulink/Logic and Bit Operations/Compare To Constant  relop===  const="fi(0,1,32,0,\"hex\",\"00000000\")"  OutDataTypeStr=boolean
  i_Genvar0_0 : Constant  Value=0  OutDataTypeStr=int32  SampleTime=-1
  i_Genvar0_1 : Constant  OutDataTypeStr=int32  SampleTime=-1
  i_Genvar0_2 : Constant  Value=2  OutDataTypeStr=int32  SampleTime=-1
  i_Genvar0_3 : Constant  Value=3  OutDataTypeStr=int32  SampleTime=-1
  sum : Outport  OutDataTypeStr=fixdt(0, 4, 0)  SampleTime=-1
  c_out : Outport  Port=2  OutDataTypeStr=fixdt(0, 1, 0)  SampleTime=-1
  wires:
  i_Genvar0_2/1 -> genblk12RelEQ80/1
  i_Genvar0_0/1 -> genblk10RelEQ80/1
  genblk10RelEQ80/1 -> Ternary/2
  Reduce_AND/1 -> Ternary_4/2
  a/1 -> Bit_Slice_6/1, Bit_Slice_4/1, Bit_Slice/1, Bit_XOR/1, Bit_Slice_2/1
  b/1 -> Bit_Slice_3/1, Bit_Slice_5/1, Bit_XOR/2, Bit_Slice_1/1, Bit_Slice_7/1
  c_in/1 -> Ternary_3/1, Ternary_2/1, Ternary_1/1, Ternary/1, Ternary_4/1
  i_Genvar0_1/1 -> genblk11RelEQ80/1
  Bit_XOR/1 -> Reduce_AND/1
  full_adder03/1(sum) -> Concat/1
  CONST_u1b_0/1 -> Ternary/3
  Bit_Slice/1 -> full_adder0/1(a)
  Bit_Slice_1/1 -> full_adder0/2(b)
  Ternary/1 -> full_adder0/3(c_in)
  Bit_Slice_6/1 -> full_adder03/1(a)
  Bit_Slice_3/1 -> full_adder01/2(b)
  genblk11RelEQ80/1 -> Ternary_1/2
  full_adder0/1(sum) -> Concat/4
  full_adder0/2(c_out) -> Ternary_1/3
  Bit_Slice_2/1 -> full_adder01/1(a)
  Ternary_1/1 -> full_adder01/3(c_in)
  Bit_Slice_5/1 -> full_adder02/2(b)
  genblk12RelEQ80/1 -> Ternary_2/2
  Ternary_4/1 -> c_out/1
  full_adder01/1(sum) -> Concat/3
  full_adder01/2(c_out) -> Ternary_2/3
  Concat/1 -> sum/1
  i_Genvar0_3/1 -> genblk13RelEQ80/1
  Bit_Slice_4/1 -> full_adder02/1(a)
  Ternary_2/1 -> full_adder02/3(c_in)
  genblk13RelEQ80/1 -> Ternary_3/2
  full_adder02/1(sum) -> Concat/2
  full_adder02/2(c_out) -> Ternary_3/3
  Bit_Slice_7/1 -> full_adder03/2(b)
  Ternary_3/1 -> full_adder03/3(c_in)
  full_adder03/2(c_out) -> Ternary_4/3

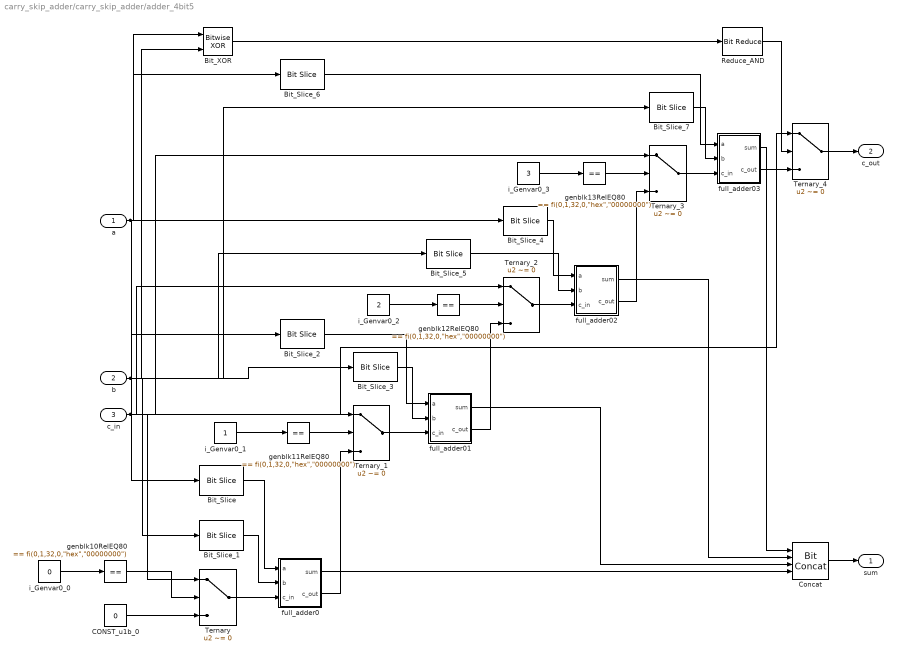
== system carry_skip_adder/carry_skip_adder/adder_4bit5 ==
  a : Inport  OutDataTypeStr=fixdt(0, 4, 0)  SampleTime=-1
  b : Inport  Port=2  OutDataTypeStr=fixdt(0, 4, 0)  SampleTime=-1
  c_in : Inport  Port=3  OutDataTypeStr=fixdt(0, 1, 0)  SampleTime=-1
  Bit_Slice : hdlsllib/Logic and Bit Operations/Bit Slice  lidx=double(0)  ridx=double(0)
  Bit_Slice_1 : hdlsllib/Logic and Bit Operations/Bit Slice  lidx=double(0)  ridx=double(0)
  Bit_Slice_2 : hdlsllib/Logic and Bit Operations/Bit Slice  lidx=double(1)  ridx=double(1)
  Bit_Slice_3 : hdlsllib/Logic and Bit Operations/Bit Slice  lidx=double(1)  ridx=double(1)
  Bit_Slice_4 : hdlsllib/Logic and Bit Operations/Bit Slice  lidx=double(2)  ridx=double(2)
  Bit_Slice_5 : hdlsllib/Logic and Bit Operations/Bit Slice  lidx=double(2)  ridx=double(2)
  Bit_Slice_6 : hdlsllib/Logic and Bit Operations/Bit Slice  lidx=double(3)  ridx=double(3)
  Bit_Slice_7 : hdlsllib/Logic and Bit Operations/Bit Slice  lidx=double(3)  ridx=double(3)
  Bit_XOR : simulink/Logic and Bit Operations/Bitwise Operator  logicop=XOR  UseBitMask=off  NumInputPorts=2  BitMask=double(0)  BitMaskRealWorld=Real World Value
  CONST_u1b_0 : Constant  Value=0  OutDataTypeStr=fixdt(0, 1, 0)  SampleTime=-1
  Concat : hdlsllib/Logic and Bit Operations/Bit Concat  numInputs=4
  Reduce_AND : hdlsllib/Logic and Bit Operations/Bit Reduce  mode=AND
  Ternary : Switch  Criteria=u2 ~= 0  Threshold=double(0)  OutDataTypeStr=fixdt(0, 1, 0)  SampleTime=-1  SaturateOnIntegerOverflow=off  InputSameDT=off
  Ternary_{1..4} (4 alike) : Switch  Criteria=u2 ~= 0  Threshold=double(0)  OutDataTypeStr=fixdt(0, 1, 0)  SampleTime=-1  SaturateOnIntegerOverflow=off  InputSameDT=off
  full_adder0 : Subsystem
  full_adder01 : Subsystem
  full_adder02 : Subsystem
  full_adder03 : Subsystem
  genblk10RelEQ80 : simulink/Logic and Bit Operations/Compare To Constant  relop===  const="fi(0,1,32,0,\"hex\",\"00000000\")"  OutDataTypeStr=boolean
  genblk11RelEQ80 : simulink/Logic and Bit Operations/Compare To Constant  relop===  const="fi(0,1,32,0,\"hex\",\"00000000\")"  OutDataTypeStr=boolean
  genblk12RelEQ80 : simulink/Logic and Bit Operations/Compare To Constant  relop===  const="fi(0,1,32,0,\"hex\",\"00000000\")"  OutDataTypeStr=boolean
  genblk13RelEQ80 : simulink/Logic and Bit Operations/Compare To Constant  relop===  const="fi(0,1,32,0,\"hex\",\"00000000\")"  OutDataTypeStr=boolean
  i_Genvar0_0 : Constant  Value=0  OutDataTypeStr=int32  SampleTime=-1
  i_Genvar0_1 : Constant  OutDataTypeStr=int32  SampleTime=-1
  i_Genvar0_2 : Constant  Value=2  OutDataTypeStr=int32  SampleTime=-1
  i_Genvar0_3 : Constant  Value=3  OutDataTypeStr=int32  SampleTime=-1
  sum : Outport  OutDataTypeStr=fixdt(0, 4, 0)  SampleTime=-1
  c_out : Outport  Port=2  OutDataTypeStr=fixdt(0, 1, 0)  SampleTime=-1
  wires:
  full_adder03/1(sum) -> Concat/1
  i_Genvar0_0/1 -> genblk10RelEQ80/1
  a/1 -> Bit_Slice_6/1, Bit_Slice_2/1, Bit_Slice_4/1, Bit_XOR/1, Bit_Slice/1
  genblk10RelEQ80/1 -> Ternary/2
  b/1 -> Bit_Slice_5/1, Bit_Slice_3/1, Bit_Slice_1/1, Bit_XOR/2, Bit_Slice_7/1
  full_adder01/2(c_out) -> Ternary_2/3
  i_Genvar0_1/1 -> genblk11RelEQ80/1
  CONST_u1b_0/1 -> Ternary/3
  c_in/1 -> Ternary_4/1, Ternary_1/1, Ternary/1, Ternary_2/1, Ternary_3/1
  Bit_XOR/1 -> Reduce_AND/1
  Bit_Slice/1 -> full_adder0/1(a)
  Bit_Slice_1/1 -> full_adder0/2(b)
  i_Genvar0_2/1 -> genblk12RelEQ80/1
  Ternary/1 -> full_adder0/3(c_in)
  Bit_Slice_6/1 -> full_adder03/1(a)
  Bit_Slice_2/1 -> full_adder01/1(a)
  genblk11RelEQ80/1 -> Ternary_1/2
  genblk12RelEQ80/1 -> Ternary_2/2
  full_adder0/1(sum) -> Concat/4
  full_adder0/2(c_out) -> Ternary_1/3
  Bit_Slice_3/1 -> full_adder01/2(b)
  Ternary_1/1 -> full_adder01/3(c_in)
  Bit_Slice_5/1 -> full_adder02/2(b)
  Reduce_AND/1 -> Ternary_4/2
  Ternary_2/1 -> full_adder02/3(c_in)
  full_adder01/1(sum) -> Concat/3
  i_Genvar0_3/1 -> genblk13RelEQ80/1
  Bit_Slice_4/1 -> full_adder02/1(a)
  genblk13RelEQ80/1 -> Ternary_3/2
  full_adder02/1(sum) -> Concat/2
  full_adder02/2(c_out) -> Ternary_3/3
  Bit_Slice_7/1 -> full_adder03/2(b)
  Ternary_3/1 -> full_adder03/3(c_in)
  full_adder03/2(c_out) -> Ternary_4/3
  Concat/1 -> sum/1
  Ternary_4/1 -> c_out/1

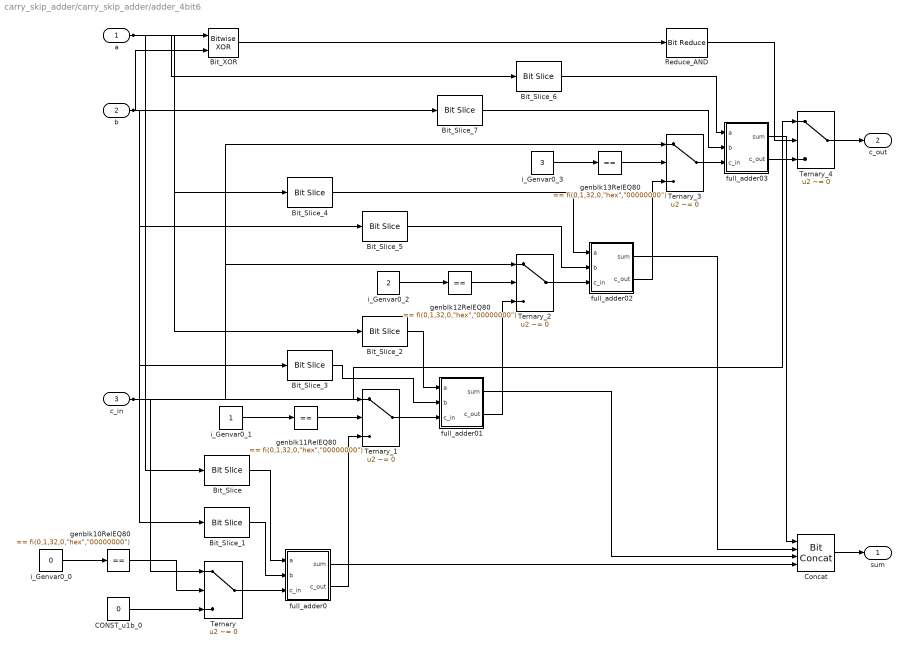
== system carry_skip_adder/carry_skip_adder/adder_4bit6 ==
  a : Inport  OutDataTypeStr=fixdt(0, 4, 0)  SampleTime=-1
  b : Inport  Port=2  OutDataTypeStr=fixdt(0, 4, 0)  SampleTime=-1
  c_in : Inport  Port=3  OutDataTypeStr=fixdt(0, 1, 0)  SampleTime=-1
  Bit_Slice : hdlsllib/Logic and Bit Operations/Bit Slice  lidx=double(0)  ridx=double(0)
  Bit_Slice_1 : hdlsllib/Logic and Bit Operations/Bit Slice  lidx=double(0)  ridx=double(0)
  Bit_Slice_2 : hdlsllib/Logic and Bit Operations/Bit Slice  lidx=double(1)  ridx=double(1)
  Bit_Slice_3 : hdlsllib/Logic and Bit Operations/Bit Slice  lidx=double(1)  ridx=double(1)
  Bit_Slice_4 : hdlsllib/Logic and Bit Operations/Bit Slice  lidx=double(2)  ridx=double(2)
  Bit_Slice_5 : hdlsllib/Logic and Bit Operations/Bit Slice  lidx=double(2)  ridx=double(2)
  Bit_Slice_6 : hdlsllib/Logic and Bit Operations/Bit Slice  lidx=double(3)  ridx=double(3)
  Bit_Slice_7 : hdlsllib/Logic and Bit Operations/Bit Slice  lidx=double(3)  ridx=double(3)
  Bit_XOR : simulink/Logic and Bit Operations/Bitwise Operator  logicop=XOR  UseBitMask=off  NumInputPorts=2  BitMask=double(0)  BitMaskRealWorld=Real World Value
  CONST_u1b_0 : Constant  Value=0  OutDataTypeStr=fixdt(0, 1, 0)  SampleTime=-1
  Concat : hdlsllib/Logic and Bit Operations/Bit Concat  numInputs=4
  Reduce_AND : hdlsllib/Logic and Bit Operations/Bit Reduce  mode=AND
  Ternary : Switch  Criteria=u2 ~= 0  Threshold=double(0)  OutDataTypeStr=fixdt(0, 1, 0)  SampleTime=-1  SaturateOnIntegerOverflow=off  InputSameDT=off
  Ternary_{1..4} (4 alike) : Switch  Criteria=u2 ~= 0  Threshold=double(0)  OutDataTypeStr=fixdt(0, 1, 0)  SampleTime=-1  SaturateOnIntegerOverflow=off  InputSameDT=off
  full_adder0 : Subsystem
  full_adder01 : Subsystem
  full_adder02 : Subsystem
  full_adder03 : Subsystem
  genblk10RelEQ80 : simulink/Logic and Bit Operations/Compare To Constant  relop===  const="fi(0,1,32,0,\"hex\",\"00000000\")"  OutDataTypeStr=boolean
  genblk11RelEQ80 : simulink/Logic and Bit Operations/Compare To Constant  relop===  const="fi(0,1,32,0,\"hex\",\"00000000\")"  OutDataTypeStr=boolean
  genblk12RelEQ80 : simulink/Logic and Bit Operations/Compare To Constant  relop===  const="fi(0,1,32,0,\"hex\",\"00000000\")"  OutDataTypeStr=boolean
  genblk13RelEQ80 : simulink/Logic and Bit Operations/Compare To Constant  relop===  const="fi(0,1,32,0,\"hex\",\"00000000\")"  OutDataTypeStr=boolean
  i_Genvar0_0 : Constant  Value=0  OutDataTypeStr=int32  SampleTime=-1
  i_Genvar0_1 : Constant  OutDataTypeStr=int32  SampleTime=-1
  i_Genvar0_2 : Constant  Value=2  OutDataTypeStr=int32  SampleTime=-1
  i_Genvar0_3 : Constant  Value=3  OutDataTypeStr=int32  SampleTime=-1
  sum : Outport  OutDataTypeStr=fixdt(0, 4, 0)  SampleTime=-1
  c_out : Outport  Port=2  OutDataTypeStr=fixdt(0, 1, 0)  SampleTime=-1
  wires:
  i_Genvar0_0/1 -> genblk10RelEQ80/1
  a/1 -> Bit_Slice_6/1, Bit_Slice_2/1, Bit_Slice/1, Bit_Slice_4/1, Bit_XOR/1
  genblk10RelEQ80/1 -> Ternary/2
  b/1 -> Bit_Slice_5/1, Bit_Slice_3/1, Bit_Slice_1/1, Bit_XOR/2, Bit_Slice_7/1
  Bit_XOR/1 -> Reduce_AND/1
  Ternary_4/1 -> c_out/1
  full_adder03/1(sum) -> Concat/1
  c_in/1 -> Ternary_4/1, Ternary_2/1, Ternary_1/1, Ternary/1, Ternary_3/1
  CONST_u1b_0/1 -> Ternary/3
  i_Genvar0_1/1 -> genblk11RelEQ80/1
  Bit_Slice/1 -> full_adder0/1(a)
  Bit_Slice_1/1 -> full_adder0/2(b)
  i_Genvar0_2/1 -> genblk12RelEQ80/1
  Ternary/1 -> full_adder0/3(c_in)
  Bit_Slice_4/1 -> full_adder02/1(a)
  Bit_Slice_3/1 -> full_adder01/2(b)
  genblk11RelEQ80/1 -> Ternary_1/2
  Bit_Slice_7/1 -> full_adder03/2(b)
  full_adder0/1(sum) -> Concat/4
  full_adder0/2(c_out) -> Ternary_1/3
  Bit_Slice_5/1 -> full_adder02/2(b)
  Bit_Slice_2/1 -> full_adder01/1(a)
  Ternary_1/1 -> full_adder01/3(c_in)
  genblk12RelEQ80/1 -> Ternary_2/2
  Concat/1 -> sum/1
  full_adder01/1(sum) -> Concat/3
  full_adder01/2(c_out) -> Ternary_2/3
  genblk13RelEQ80/1 -> Ternary_3/2
  Bit_Slice_6/1 -> full_adder03/1(a)
  i_Genvar0_3/1 -> genblk13RelEQ80/1
  Reduce_AND/1 -> Ternary_4/2
  Ternary_2/1 -> full_adder02/3(c_in)
  full_adder02/1(sum) -> Concat/2
  full_adder02/2(c_out) -> Ternary_3/3
  Ternary_3/1 -> full_adder03/3(c_in)
  full_adder03/2(c_out) -> Ternary_4/3

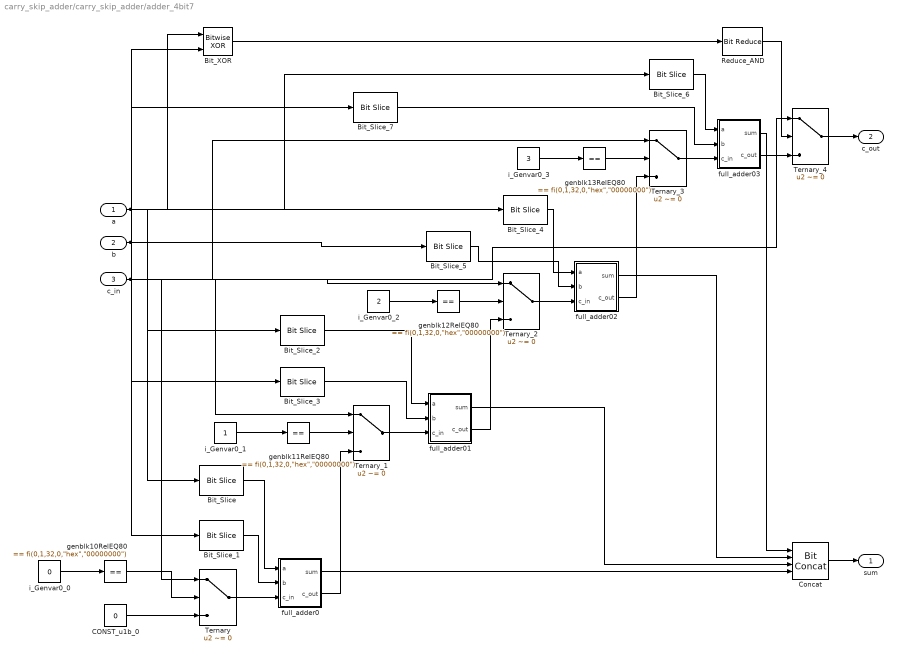
== system carry_skip_adder/carry_skip_adder/adder_4bit7 ==
  a : Inport  OutDataTypeStr=fixdt(0, 4, 0)  SampleTime=-1
  b : Inport  Port=2  OutDataTypeStr=fixdt(0, 4, 0)  SampleTime=-1
  c_in : Inport  Port=3  OutDataTypeStr=fixdt(0, 1, 0)  SampleTime=-1
  Bit_Slice : hdlsllib/Logic and Bit Operations/Bit Slice  lidx=double(0)  ridx=double(0)
  Bit_Slice_1 : hdlsllib/Logic and Bit Operations/Bit Slice  lidx=double(0)  ridx=double(0)
  Bit_Slice_2 : hdlsllib/Logic and Bit Operations/Bit Slice  lidx=double(1)  ridx=double(1)
  Bit_Slice_3 : hdlsllib/Logic and Bit Operations/Bit Slice  lidx=double(1)  ridx=double(1)
  Bit_Slice_4 : hdlsllib/Logic and Bit Operations/Bit Slice  lidx=double(2)  ridx=double(2)
  Bit_Slice_5 : hdlsllib/Logic and Bit Operations/Bit Slice  lidx=double(2)  ridx=double(2)
  Bit_Slice_6 : hdlsllib/Logic and Bit Operations/Bit Slice  lidx=double(3)  ridx=double(3)
  Bit_Slice_7 : hdlsllib/Logic and Bit Operations/Bit Slice  lidx=double(3)  ridx=double(3)
  Bit_XOR : simulink/Logic and Bit Operations/Bitwise Operator  logicop=XOR  UseBitMask=off  NumInputPorts=2  BitMask=double(0)  BitMaskRealWorld=Real World Value
  CONST_u1b_0 : Constant  Value=0  OutDataTypeStr=fixdt(0, 1, 0)  SampleTime=-1
  Concat : hdlsllib/Logic and Bit Operations/Bit Concat  numInputs=4
  Reduce_AND : hdlsllib/Logic and Bit Operations/Bit Reduce  mode=AND
  Ternary : Switch  Criteria=u2 ~= 0  Threshold=double(0)  OutDataTypeStr=fixdt(0, 1, 0)  SampleTime=-1  SaturateOnIntegerOverflow=off  InputSameDT=off
  Ternary_{1..4} (4 alike) : Switch  Criteria=u2 ~= 0  Threshold=double(0)  OutDataTypeStr=fixdt(0, 1, 0)  SampleTime=-1  SaturateOnIntegerOverflow=off  InputSameDT=off
  full_adder0 : Subsystem
  full_adder01 : Subsystem
  full_adder02 : Subsystem
  full_adder03 : Subsystem
  genblk10RelEQ80 : simulink/Logic and Bit Operations/Compare To Constant  relop===  const="fi(0,1,32,0,\"hex\",\"00000000\")"  OutDataTypeStr=boolean
  genblk11RelEQ80 : simulink/Logic and Bit Operations/Compare To Constant  relop===  const="fi(0,1,32,0,\"hex\",\"00000000\")"  OutDataTypeStr=boolean
  genblk12RelEQ80 : simulink/Logic and Bit Operations/Compare To Constant  relop===  const="fi(0,1,32,0,\"hex\",\"00000000\")"  OutDataTypeStr=boolean
  genblk13RelEQ80 : simulink/Logic and Bit Operations/Compare To Constant  relop===  const="fi(0,1,32,0,\"hex\",\"00000000\")"  OutDataTypeStr=boolean
  i_Genvar0_0 : Constant  Value=0  OutDataTypeStr=int32  SampleTime=-1
  i_Genvar0_1 : Constant  OutDataTypeStr=int32  SampleTime=-1
  i_Genvar0_2 : Constant  Value=2  OutDataTypeStr=int32  SampleTime=-1
  i_Genvar0_3 : Constant  Value=3  OutDataTypeStr=int32  SampleTime=-1
  sum : Outport  OutDataTypeStr=fixdt(0, 4, 0)  SampleTime=-1
  c_out : Outport  Port=2  OutDataTypeStr=fixdt(0, 1, 0)  SampleTime=-1
  wires:
  Ternary_1/1 -> full_adder01/3(c_in)
  i_Genvar0_0/1 -> genblk10RelEQ80/1
  genblk12RelEQ80/1 -> Ternary_2/2
  genblk10RelEQ80/1 -> Ternary/2
  Reduce_AND/1 -> Ternary_4/2
  a/1 -> Bit_Slice_2/1, Bit_Slice/1, Bit_Slice_4/1, Bit_XOR/1, Bit_Slice_6/1
  b/1 -> Bit_Slice_7/1, Bit_Slice_5/1, Bit_Slice_1/1, Bit_XOR/2, Bit_Slice_3/1
  c_in/1 -> Ternary_4/1, Ternary_2/1, Ternary_1/1, Ternary_3/1, Ternary/1
  CONST_u1b_0/1 -> Ternary/3
  Bit_XOR/1 -> Reduce_AND/1
  i_Genvar0_1/1 -> genblk11RelEQ80/1
  Bit_Slice/1 -> full_adder0/1(a)
  i_Genvar0_3/1 -> genblk13RelEQ80/1
  Bit_Slice_1/1 -> full_adder0/2(b)
  Bit_Slice_2/1 -> full_adder01/1(a)
  Ternary/1 -> full_adder0/3(c_in)
  Bit_Slice_3/1 -> full_adder01/2(b)
  genblk11RelEQ80/1 -> Ternary_1/2
  full_adder0/1(sum) -> Concat/4
  full_adder0/2(c_out) -> Ternary_1/3
  Bit_Slice_7/1 -> full_adder03/2(b)
  full_adder02/1(sum) -> Concat/2
  i_Genvar0_2/1 -> genblk12RelEQ80/1
  Bit_Slice_5/1 -> full_adder02/2(b)
  full_adder01/1(sum) -> Concat/3
  full_adder01/2(c_out) -> Ternary_2/3
  Bit_Slice_4/1 -> full_adder02/1(a)
  Ternary_2/1 -> full_adder02/3(c_in)
  genblk13RelEQ80/1 -> Ternary_3/2
  full_adder02/2(c_out) -> Ternary_3/3
  Bit_Slice_6/1 -> full_adder03/1(a)
  Ternary_3/1 -> full_adder03/3(c_in)
  full_adder03/1(sum) -> Concat/1
  full_adder03/2(c_out) -> Ternary_4/3
  Ternary_4/1 -> c_out/1
  Concat/1 -> sum/1

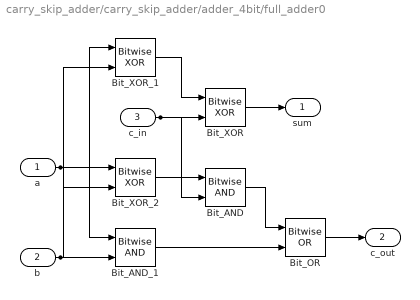
== system carry_skip_adder/carry_skip_adder/adder_4bit/full_adder0 ==
  a : Inport  OutDataTypeStr=fixdt(0, 1, 0)  SampleTime=-1
  b : Inport  Port=2  OutDataTypeStr=fixdt(0, 1, 0)  SampleTime=-1
  c_in : Inport  Port=3  OutDataTypeStr=fixdt(0, 1, 0)  SampleTime=-1
  Bit_AND : simulink/Logic and Bit Operations/Bitwise Operator  logicop=AND  UseBitMask=off  NumInputPorts=2  BitMask=double(0)  BitMaskRealWorld=Real World Value
  Bit_AND_1 : simulink/Logic and Bit Operations/Bitwise Operator  logicop=AND  UseBitMask=off  NumInputPorts=2  BitMask=double(0)  BitMaskRealWorld=Real World Value
  Bit_OR : simulink/Logic and Bit Operations/Bitwise Operator  logicop=OR  UseBitMask=off  NumInputPorts=2  BitMask=double(0)  BitMaskRealWorld=Real World Value
  Bit_XOR : simulink/Logic and Bit Operations/Bitwise Operator  logicop=XOR  UseBitMask=off  NumInputPorts=2  BitMask=double(0)  BitMaskRealWorld=Real World Value
  Bit_XOR_1 : simulink/Logic and Bit Operations/Bitwise Operator  logicop=XOR  UseBitMask=off  NumInputPorts=2  BitMask=double(0)  BitMaskRealWorld=Real World Value
  Bit_XOR_2 : simulink/Logic and Bit Operations/Bitwise Operator  logicop=XOR  UseBitMask=off  NumInputPorts=2  BitMask=double(0)  BitMaskRealWorld=Real World Value
  sum : Outport  OutDataTypeStr=fixdt(0, 1, 0)  SampleTime=-1
  c_out : Outport  Port=2  OutDataTypeStr=fixdt(0, 1, 0)  SampleTime=-1
  wires:
  a/1 -> Bit_AND_1/1, Bit_XOR_2/1, Bit_XOR_1/1
  b/1 -> Bit_AND_1/2, Bit_XOR_2/2, Bit_XOR_1/2
  Bit_AND/1 -> Bit_OR/1
  Bit_XOR/1 -> sum/1
  Bit_AND_1/1 -> Bit_OR/2
  Bit_XOR_2/1 -> Bit_AND/1
  Bit_XOR_1/1 -> Bit_XOR/1
  c_in/1 -> Bit_AND/2, Bit_XOR/2
  Bit_OR/1 -> c_out/1

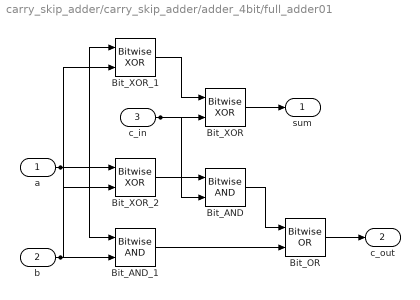
== system carry_skip_adder/carry_skip_adder/adder_4bit/full_adder01 ==
  a : Inport  OutDataTypeStr=fixdt(0, 1, 0)  SampleTime=-1
  b : Inport  Port=2  OutDataTypeStr=fixdt(0, 1, 0)  SampleTime=-1
  c_in : Inport  Port=3  OutDataTypeStr=fixdt(0, 1, 0)  SampleTime=-1
  Bit_AND : simulink/Logic and Bit Operations/Bitwise Operator  logicop=AND  UseBitMask=off  NumInputPorts=2  BitMask=double(0)  BitMaskRealWorld=Real World Value
  Bit_AND_1 : simulink/Logic and Bit Operations/Bitwise Operator  logicop=AND  UseBitMask=off  NumInputPorts=2  BitMask=double(0)  BitMaskRealWorld=Real World Value
  Bit_OR : simulink/Logic and Bit Operations/Bitwise Operator  logicop=OR  UseBitMask=off  NumInputPorts=2  BitMask=double(0)  BitMaskRealWorld=Real World Value
  Bit_XOR : simulink/Logic and Bit Operations/Bitwise Operator  logicop=XOR  UseBitMask=off  NumInputPorts=2  BitMask=double(0)  BitMaskRealWorld=Real World Value
  Bit_XOR_1 : simulink/Logic and Bit Operations/Bitwise Operator  logicop=XOR  UseBitMask=off  NumInputPorts=2  BitMask=double(0)  BitMaskRealWorld=Real World Value
  Bit_XOR_2 : simulink/Logic and Bit Operations/Bitwise Operator  logicop=XOR  UseBitMask=off  NumInputPorts=2  BitMask=double(0)  BitMaskRealWorld=Real World Value
  sum : Outport  OutDataTypeStr=fixdt(0, 1, 0)  SampleTime=-1
  c_out : Outport  Port=2  OutDataTypeStr=fixdt(0, 1, 0)  SampleTime=-1
  wires:
  a/1 -> Bit_AND_1/1, Bit_XOR_2/1, Bit_XOR_1/1
  b/1 -> Bit_AND_1/2, Bit_XOR_2/2, Bit_XOR_1/2
  Bit_AND/1 -> Bit_OR/1
  Bit_XOR/1 -> sum/1
  Bit_AND_1/1 -> Bit_OR/2
  Bit_XOR_2/1 -> Bit_AND/1
  Bit_XOR_1/1 -> Bit_XOR/1
  c_in/1 -> Bit_AND/2, Bit_XOR/2
  Bit_OR/1 -> c_out/1

== system carry_skip_adder/carry_skip_adder/adder_4bit/full_adder02 ==
  a : Inport  OutDataTypeStr=fixdt(0, 1, 0)  SampleTime=-1
  b : Inport  Port=2  OutDataTypeStr=fixdt(0, 1, 0)  SampleTime=-1
  c_in : Inport  Port=3  OutDataTypeStr=fixdt(0, 1, 0)  SampleTime=-1
  Bit_AND : simulink/Logic and Bit Operations/Bitwise Operator  logicop=AND  UseBitMask=off  NumInputPorts=2  BitMask=double(0)  BitMaskRealWorld=Real World Value
  Bit_AND_1 : simulink/Logic and Bit Operations/Bitwise Operator  logicop=AND  UseBitMask=off  NumInputPorts=2  BitMask=double(0)  BitMaskRealWorld=Real World Value
  Bit_OR : simulink/Logic and Bit Operations/Bitwise Operator  logicop=OR  UseBitMask=off  NumInputPorts=2  BitMask=double(0)  BitMaskRealWorld=Real World Value
  Bit_XOR : simulink/Logic and Bit Operations/Bitwise Operator  logicop=XOR  UseBitMask=off  NumInputPorts=2  BitMask=double(0)  BitMaskRealWorld=Real World Value
  Bit_XOR_1 : simulink/Logic and Bit Operations/Bitwise Operator  logicop=XOR  UseBitMask=off  NumInputPorts=2  BitMask=double(0)  BitMaskRealWorld=Real World Value
  Bit_XOR_2 : simulink/Logic and Bit Operations/Bitwise Operator  logicop=XOR  UseBitMask=off  NumInputPorts=2  BitMask=double(0)  BitMaskRealWorld=Real World Value
  sum : Outport  OutDataTypeStr=fixdt(0, 1, 0)  SampleTime=-1
  c_out : Outport  Port=2  OutDataTypeStr=fixdt(0, 1, 0)  SampleTime=-1
  wires:
  Bit_AND/1 -> Bit_OR/1
  a/1 -> Bit_AND_1/1, Bit_XOR_2/1, Bit_XOR_1/1
  Bit_XOR/1 -> sum/1
  Bit_AND_1/1 -> Bit_OR/2
  Bit_XOR_2/1 -> Bit_AND/1
  Bit_XOR_1/1 -> Bit_XOR/1
  b/1 -> Bit_AND_1/2, Bit_XOR_1/2, Bit_XOR_2/2
  c_in/1 -> Bit_XOR/2, Bit_AND/2
  Bit_OR/1 -> c_out/1
